simulink model "PMSM_DemoBackup"  (R2020a)
settings: Solver=FixedStepDiscrete  StartTime=0.0  StopTime=Inf  FixedStep=1000e-6  RelTol=1e-3  EnableMultiTasking=on
PreLoadFcn:
  | run('PMSM_Demo_ini.m');
PostLoadFcn:
  | , if any(exist('dsrtsu_mdlpostloadfcn', 'file') ~= 0), dsrtsu_mdlpostloadfcn('Execute', bdroot); end,
InitFcn:
  | , if any(exist('rtifpga_mdlclblib', 'file') ~= 0), rtifpga_mdlclblib('Init', bdroot); end,
undefined symbols (not defined in the file): clock, Const_Id_Fieldweakening, Const_Ld_Stator, Const_Lq_Stator, Const_PolePairs, Const_Psi, Newton, PMSM_Ctrl_Ctrl_mode_SW, PMSM_Ctrl_fRS_Set, PMSM_Ctrl_i_d_Set, PMSM_Ctrl_i_d_Stroke, PMSM_Ctrl_i_q_Set, PMSM_Ctrl_i_q_Stroke, PMSM_Ctrl_Ki_id, PMSM_Ctrl_Ki_iq, PMSM_Ctrl_Ki_n, PMSM_Ctrl_Kp_id, PMSM_Ctrl_Kp_iq, PMSM_Ctrl_Kp_n, PMSM_Ctrl_Limit_iq, PMSM_Ctrl_load_torque, PMSM_Ctrl_n_Limit, PMSM_Ctrl_n_Set, PMSM_Ctrl_n_Stroke, PMSM_Ctrl_Pos_Src, PMSM_Ctrl_TF_Id, PMSM_Ctrl_TF_Iq, PMSM_Ctrl_TF_n, PMSM_Ctrl_theta_offset, PMSM_Ctrl_v_d_Set, PMSM_Ctrl_V_DCLink_Limit, PMSM_Ctrl_v_q_Set, PMSM_Ctrl_Vel_Src, Raphson, rpm_to_rad, s, SW_Fieldweakening, T_PWM
libraries: simulink x37, rti1202lib_adc_class1 x8, dsextras x4, rtiemclib x4, rti1202lib_dio_class1 x3, ASM_ElectricComponents_lib x2, ASM_Utils_lib x1, rti1202lib_base x1
(part 2 of 4)

== system PMSM_DemoBackup/Control/Output ==
  note: a,b,c
      | a,c,b
      | b,a,c
      | b,c,a
      | c,a,b
      | c,b,a
  T_Sample[s] : Inport
  PWM_Duty[a,b,c] : Inport  Port=2
  Bus Selector : BusSelector  OutputSignals=DutyCycle[a;b;c][HSD].DutyCycle_a_HSD[0_1],DutyCycle[a;b;c][HSD].DutyCycle_b_HSD[0_1],DutyCycle[a;b;c][HSD].DutyCycle_c_HSD[0_1]
  Duty_A : Constant  Value=0
  Duty_B : Constant  Value=0
  Duty_C : Constant  Value=0
  EMC_MC_PWM_BL1 : rtiemclib/EMC_MC_PWM_BL1  DSProperties=struct('RTI',struct('Version',uint32(2),'BlockType',struct('isSLSource',uint8(0),'isSLSink',uint8(1),'isHWSource',uint8(0),'isHWSink',uint8(1),'isSetup',uint8(0),'isInline',uint8(1),'isNonInline',uint8(0),'isInterrupt',uint8(0),'isChannelwise',uint8(1)),'IOBoardType','DSEMC','UnitType','MCPWM','Identifier','MCPWM','DialogType','ML','BlockSet','RTIEMC','SlaveProcessor','NONE'))  RTIBlockInterface=struct('InputPortsWidth',int32([1 3 1]),'InputPortsActive',[1 1 0],'InputPortsName',{{'Period',['Duty Cycle'],['Output Enable']}},'BlockDisplay',{{['EMC Multi Channel PWM\nPort: 1\nChannel: 7\nNumber of channels: 3'],'center'}},'IconTransparency','on','InitLevel',3,'DialogFcn','rtiemcmcpwmgui','BlockName',struct('Token',{{'EMC_MC_PWM_BL1'}}),'InputPortsDataType',{{'SS_DOUBLE','SS_DOUBLE','SS_BOOLEAN'}})  RTIBlockParameters=struct('PortNo',{{1,'OFF',[1 3]}},'ChannelNo',{{7,'OFF',[1 16]}},'InvChannelMode',{{2,'OFF',[1 2]}},'NumOfChannels',{{3,'OFF',[1 5]}},'HighLevel',{{3,'OFF',[1 3]}},'AlignmentMode',{{1,'OFF',[1 2]}},'UpdateModeCA',{{3,'OFF',[1 3]}},'UpdateModeEA',{{1,'OFF',[1 2]}},'DeadTime',{{'0.000001','OFF',[0 0.000655]}},'InitPeriod',{{'5e-05','OFF',[1e-7 1.34]}},'InitDutyCycle1',{{'0.5','OFF',[0 1]}},'InitDutyCycle2',{{'0.5','OFF',[0 1]}},'InitDutyCycle3',{{'0.5','OFF',[0 1]}},'InitDutyCycle4',{{'0.5','OFF',[0 1]}},'InitDutyCycle5',{{'0.5','OFF',[0 1]}},'InitDutyCycle6',{{'0.5','OFF',[0 1]}},'InitDutyCycle7',{{'0','OFF',[0 1]}},'InitDutyCycle8',{{'0','OFF',[0 1]}},'InitDutyCycle9',{{'0','OFF',[0 1]}},'InitDutyCycle10',{{'0.5','OFF',[0 1]}},'InitDutyCycle11',{{'0.5','OFF',[0 1]}},'InitDutyCycle12',{{'0.5','OFF',[0 1]}},'InitDutyCycle13',{{'0.5','OFF',[0 1]}},'InitDutyCycle14',{{'0.5','OFF',[0 1]}},'InitDutyCycle15',{{'0.5','OFF',[0 1]}},'InitDutyCycle16',{{'0.5','OFF',[0 1]}},'TerminationMode',{{0,'OFF',[0 1]}},'OutputTermValidate',{{0,'OFF',[0 1]}},'TermPeriod',{{'5e-05','OFF',[1e-7 1.34]}},'TermDutyCycle1',{{'0.5','OFF',[0 1]}},'TermDutyCycle2',{{'0.5','OFF',[0 1]}},'TermDutyCycle3',{{'0.5','OFF',[0 1]}},'TermDutyCycle4',{{'0.5','OFF',[0 1]}},'TermDutyCycle5',{{'0.5','OFF',[0 1]}},'TermDutyCycle6',{{'0.5','OFF',[0 1]}},'TermDutyCycle7',{{'0.5','OFF',[0 1]}},'TermDutyCycle8',{{'0.5','OFF',[0 1]}},'TermDutyCycle9',{{'0.5','OFF',[0 1]}},'TermDutyCycle10',{{'0.5','OFF',[0 1]}},'TermDutyCycle11',{{'0.5','OFF',[0 1]}},'TermDutyCycle12',{{'0.5','OFF',[0 1]}},'TermDutyCycle13',{{'0.5','OFF',[0 1]}},'TermDutyCycle14',{{'0.5','OFF',[0 1]}},'TermDutyCycle15',{{'0.5','OFF',[0 1]}},'TermDutyCycle16',{{'0.5','OFF',[0 1]}},'EnableEvent',{{1,'OFF',[0 1]}},'EventMode',{{3,'OFF',[1 3]}},'EventOnStart',{{0,'OFF',[0 1]}},'EventOnCenter',{{1,'OFF',[0 1]}},'EventDelay',{{'0','OFF',[0 1.34]}},'EventRate',{{'1','OFF',[1 256]}},'TriggerLine',{{1,'OFF',[1 16]}},'TLCFileName',{{'rtiemcmcpwm','OFF',[]}},'ValidateDeadTimeBuildCheck',{{true,'OFF',[]}},'InitDutyCycleBuildCheck1',{{0,'OFF',[]}},'InitDutyCycleBuildCheck2',{{0,'OFF',[]}},'InitDutyCycleBuildCheck3',{{0,'OFF',[]}},'InitDutyCycleBuildCheck4',{{0,'OFF',[]}},'InitDutyCycleBuildCheck5',{{0,'OFF',[]}},'InitDutyCycleBuildCheck6',{{0,'OFF',[]}},'InitDutyCycleBuildCheck7',{{1,'OFF',[]}},'InitDutyCycleBuildCheck8',{{1,'OFF',[]}},'InitDutyCycleBuildCheck9',{{1,'OFF',[]}},'InitDutyCycleBuildCheck10',{{0,'OFF',[]}},'InitDutyCycleBuildCheck11',{{0,'OFF',[]}},'InitDutyCycleBuildCheck12',{{0,'OFF',[]}},'InitDutyCycleBuildCheck13',{{0,'OFF',[]}},'InitDutyCycleBuildCheck14',{{0,'OFF',[]}},'InitDutyCycleBuildCheck15',{{0,'OFF',[]}},'InitDutyCycleBuildCheck16',{{0,'OFF',[]}},'ValidateTermBuildCheck',{{false,'OFF',[]}},'TermDutyCycleBuildCheck1',{{0,'OFF',[]}},'TermDutyCycleBuildCheck2',{{0,'OFF',[]}},'TermDutyCycleBuildCheck3',{{0,'OFF',[]}},'TermDutyCycleBuildCheck4',{{0,'OFF',[]}},'TermDutyCycleBuildCheck5',{{0,'OFF',[]}},'TermDutyCycleBuildCheck6',{{0,'OFF',[]}},'TermDutyCycleBuildCheck7',{{0,'OFF',[]}},'TermDutyCycleBuildCheck8',{{0,'OFF',[]}},'TermDutyCycleBuildCheck9',{{0,'OFF',[]}},'TermDutyCycleBuildCheck10',{{0,'OFF',[]}},'TermDutyCycleBuildCheck11',{{0,'OFF',[]}},'TermDutyCycleBuildCheck12',{{0,'OFF',[]}},'TermDutyCycleBuildCheck13',{{0,'OFF',[]}},'TermDutyCycleBuildCheck14',{{0,'OFF',[]}},'TermDutyCycleBuildCheck15',{{0,'OFF',[]}},'TermDutyCycleBuildCheck16',{{0,'OFF',[]}},'ValidateEventBuildCheck',{{true,'OFF',[]}},'ActivateOutputEnablePort',{{0,'OFF',[0 1]}},'InitOutputEnable',{{1,'OFF',[1 2]}})  RTISFcnParameters=struct('PortNo','int32','ChannelNo','int32','InvChannelMode','int32','NumOfChannels','int32','HighLevel','int32','AlignmentMode','int32','UpdateModeCA','int32','UpdateModeEA','int32','DeadTime','double','InitPeriod','double','InitDutyCycle1','double','InitDutyCycle2','double','InitDutyCycle3','double','InitDutyCycle4','double','InitDutyCycle5','double','InitDutyCycle6','double','InitDutyCycle7','double','InitDutyCycle8','double','InitDutyCycle9','double','InitDutyCycle10','double','InitDutyCycle11','double','InitDutyCycle12','double','InitDutyCycle13','double','InitDutyCycle14','double','InitDutyCycle15','double','InitDutyCycle16','double','TerminationMode','uint32','OutputTermValidate','int32','TermPeriod','double','TermDutyCycle1','double','TermDutyCycle2','double','TermDutyCycle3','double','TermDutyCycle4','double','TermDutyCycle5','double','TermDutyCycle6','double','TermDutyCycle7','double','TermDutyCycle8','double','TermDutyCycle9','double','TermDutyCycle10','double','TermDutyCycle11','double','TermDutyCycle12','double','TermDutyCycle13','double','TermDutyCycle14','double','TermDutyCycle15','double','TermDutyCycle16','double','EnableEvent','int32','EventMode','int32','EventOnStart','int32','EventOnCenter','int32','EventDelay','double','EventRate','int32','TriggerLine','int32','TLCFileName','char','ActivateOutputEnablePort','int32','InitOutputEnable','int32')  RTIBlockParaDefault=struct('PortNo',1,'ChannelNo',1,'InvChannelMode',1,'NumOfChannels',1,'HighLevel',1,'AlignmentMode',1,'UpdateModeCA',1,'UpdateModeEA',1,'DeadTime',0,'InitPeriod',5e-5,'InitDutyCycle1',2^-1,'InitDutyCycle2',2^-1,'InitDutyCycle3',2^-1,'InitDutyCycle4',2^-1,'InitDutyCycle5',2^-1,'InitDutyCycle6',2^-1,'InitDutyCycle7',2^-1,'InitDutyCycle8',2^-1,'InitDutyCycle9',2^-1,'InitDutyCycle10',2^-1,'InitDutyCycle11',2^-1,'InitDutyCycle12',2^-1,'InitDutyCycle13',2^-1,'InitDutyCycle14',2^-1,'InitDutyCycle15',2^-1,'InitDutyCycle16',2^-1,'TerminationMode',0,'OutputTermValidate',0,'TermPeriod',5e-5,'TermDutyCycle1',2^-1,'TermDutyCycle2',2^-1,'TermDutyCycle3',2^-1,'TermDutyCycle4',2^-1,'TermDutyCycle5',2^-1,'TermDutyCycle6',2^-1,'TermDutyCycle7',2^-1,'TermDutyCycle8',2^-1,'TermDutyCycle9',2^-1,'TermDutyCycle10',2^-1,'TermDutyCycle11',2^-1,'TermDutyCycle12',2^-1,'TermDutyCycle13',2^-1,'TermDutyCycle14',2^-1,'TermDutyCycle15',2^-1,'TermDutyCycle16',2^-1,'EnableEvent',0,'EventMode',1,'EventOnStart',1,'EventOnCenter',0,'EventDelay',0,'EventRate',1,'TriggerLine',1,'TLCFileName','rtiemcmcpwm','ValidateDeadTimeBuildCheck',0,'InitDutyCycleBuildCheck1',0,'InitDutyCycleBuildCheck2',0,'InitDutyCycleBuildCheck3',0,'InitDutyCycleBuildCheck4',0,'InitDutyCycleBuildCheck5',0,'InitDutyCycleBuildCheck6',0,'InitDutyCycleBuildCheck7',0,'InitDutyCycleBuildCheck8',0,'InitDutyCycleBuildCheck9',0,'InitDutyCycleBuildCheck10',0,'InitDutyCycleBuildCheck11',0,'InitDutyCycleBuildCheck12',0,'InitDutyCycleBuildCheck13',0,'InitDutyCycleBuildCheck14',0,'InitDutyCycleBuildCheck15',0,'InitDutyCycleBuildCheck16',0,'ValidateTermBuildCheck',0,'TermDutyCycleBuildCheck1',0,'TermDutyCycleBuildCheck2',0,'TermDutyCycleBuildCheck3',0,'TermDutyCycleBuildCheck4',0,'TermDutyCycleBuildCheck5',0,'TermDutyCycleBuildCheck6',0,'TermDutyCycleBuildCheck7',0,'TermDutyCycleBuildCheck8',0,'TermDutyCycleBuildCheck9',0,'TermDutyCycleBuildCheck10',0,'TermDutyCycleBuildCheck11',0,'TermDutyCycleBuildCheck12',0,'TermDutyCycleBuildCheck13',0,'TermDutyCycleBuildCheck14',0,'TermDutyCycleBuildCheck15',0,'TermDutyCycleBuildCheck16',0,'ValidateEventBuildCheck',0,'ActivateOutputEnablePort',0,'InitOutputEnable',1)
      settings: SourceProductName=dSPACE RTI Electric Motor Control Blockset
  Mux : Mux  Inputs=3
  Mux1 : Mux  Inputs=3
  Switch : Switch  Criteria=u2 ~= 0
  UseController : Constant
  wires:
  PWM_Duty[a,b,c]/1 -> Bus Selector/1
  T_Sample[s]/1 -> EMC_MC_PWM_BL1/1
  Bus Selector/1 -> Mux/1  "<DutyCycle_a_HSD[0_1]>"
  Bus Selector/2 -> Mux/2  "<DutyCycle_b_HSD[0_1]>"
  Bus Selector/3 -> Mux/3  "<DutyCycle_c_HSD[0_1]>"
  Duty_A/1 -> Mux1/1
  Duty_C/1 -> Mux1/3
  Duty_B/1 -> Mux1/2
  Switch/1 -> EMC_MC_PWM_BL1/2
  Mux/1 -> Switch/1
  Mux1/1 -> Switch/3
  UseController/1 -> Switch/2

== system PMSM_DemoBackup/Control/pmsm_ctrl_par_sig ==
  rect_pulse : Inport
  MDL_DISP : Subsystem
      mask Display: disp('Simulation results:\nArbitrary input to\nControlDesk from MDL')
  MDL_DISP_INPUT : Subsystem
      mask Display: disp('Simulation results:\nArbitrary input to\nControlDesk from MDL')
  MDL_PAR : Subsystem
      mask Display: disp('Simulation parameters:\nContinuous output from\nControlDesk to MDL')
  wires:
  rect_pulse/1 -> MDL_PAR/1(rect_pulse)

== system PMSM_DemoBackup/RTI Data/RTI Data Store ==
  RTI Data Store : Subsystem  mask(RTI_DATA_STORE){}
      mask help:
      | RTI Data Store Block. This block is used by RTI to store internal model dependent data. Deleting this block will result in data loss.
      |
      | NEVER DELETE, COPY, OR MODIFY THIS BLOCK!
      mask Help:
      | RTI Data Store Block. This block is used by RTI to store internal model dependent data. Deleting this block will result in data loss.
      | 
      | NEVER DELETE, COPY, OR MODIFY THIS BLOCK!
      mask Display: text(0.5, 0.5, ' ', 'HorizontalAlignment', 'center');

== system PMSM_DemoBackup/Ref_value_gen/Enabled and Triggered Subsystem ==
  n_ref : Inport
  Constant : Constant
  Constant1 : Constant  Value=0
  Hit Crossing : HitCross  HitCrossingOffset=0.5  HitCrossingDirection=rising
  Memory : Memory  InheritSampleTime=on
  Product : Product  RndMeth=Zero
  Relational Operator : RelationalOperator  Operator=<=  OutDataTypeStr=boolean  RndMeth=Nearest
  Relational Operator1 : RelationalOperator  OutDataTypeStr=boolean  RndMeth=Nearest
  Sum : Sum  Inputs=|++
  Switch : Switch  Threshold=0.5
  Switch1 : Switch  Threshold=0.5
  load_signal_0 : Constant  Value=0
  load_signal_generator : Constant
  start_time_samples : Constant  Value=1000
  switch_out_boarder : Constant  Value=0.5
  load_ref : Outport  VectorParamsAs1DForOutWhenUnconnected=off
  wires:
  Constant/1 -> Sum/1
  Sum/1 -> Switch/3
  Constant1/1 -> Switch/1
  Switch/1 -> Relational Operator/1, Memory/1
  Hit Crossing/1 -> Switch/2
  n_ref/1 -> Hit Crossing/1, Relational Operator1/1
  start_time_samples/1 -> Relational Operator/2
  load_signal_0/1 -> Switch1/1
  Relational Operator/1 -> Switch1/2
  load_signal_generator/1 -> Switch1/3
  Switch1/1 -> Product/2
  switch_out_boarder/1 -> Relational Operator1/2
  Product/1 -> load_ref/1
  Relational Operator1/1 -> Product/1
  Memory/1 -> Sum/2

== system PMSM_DemoBackup/Control/Control_load_machine/duty_cycle_2_torque ==
  In_duty_cycle[0..1] : Inport
  Divide : Product  Inputs=*/
  coil_resistance : Constant  Value=24
  current_2_load1 : Lookup_n-D  NumberOfTableDimensions=1  BreakpointsForDimension1=[0, 0.05, 0.1, 0.2, 0.3, 0.4]  Table=[0, 0.05, 0.2, 0.7, 1.4, 1.9]  InputSameDT=on
  duty_cycle_2_voltage : Subsystem
  Out_torque[Nm] : Outport  VectorParamsAs1DForOutWhenUnconnected=off
  wires:
  In_duty_cycle[0..1]/1 -> duty_cycle_2_voltage/1(In_duty_cycle[0..1])
  duty_cycle_2_voltage/1(Out_duty_voltage[V]) -> Divide/1
  coil_resistance/1 -> Divide/2
  current_2_load1/1 -> Out_torque[Nm]/1
  Divide/1 -> current_2_load1/1

== system PMSM_DemoBackup/Control/Control_load_machine/torque_2_duty_cycle ==
  In_torque[Nm] : Inport
  current_2_voltage : Gain  Gain=24
  load_2_current4 : Lookup_n-D  NumberOfTableDimensions=1  BreakpointsForDimension1=[0, 0.05, 0.2, 0.7, 1.4, 1.9]  Table=[0, 0.05, 0.1, 0.2, 0.3, 0.4]  InputSameDT=on
  voltage_2_duty_cycle : Subsystem
  Out_duty_cycle[0..1] : Outport  VectorParamsAs1DForOutWhenUnconnected=off
  wires:
  load_2_current4/1 -> current_2_voltage/1
  current_2_voltage/1 -> voltage_2_duty_cycle/1(In_voltage[V])
  In_torque[Nm]/1 -> load_2_current4/1
  voltage_2_duty_cycle/1(Out_duty_cycle) -> Out_duty_cycle[0..1]/1

== system PMSM_DemoBackup/Control/Control_load_machine/torque_2_duty_cycle1 ==
  In_torque[Nm] : Inport
  current_2_voltage : Gain  Gain=24
  load_2_current4 : Lookup_n-D  NumberOfTableDimensions=1  BreakpointsForDimension1=[0, 0.05, 0.2, 0.7, 1.4, 1.9]  Table=[0, 0.05, 0.1, 0.2, 0.3, 0.4]  InputSameDT=on
  voltage_2_duty_cycle : Subsystem
  Out_duty_cycle[0..1] : Outport  VectorParamsAs1DForOutWhenUnconnected=off
  wires:
  voltage_2_duty_cycle/1(Out_duty_cycle[0..1]) -> Out_duty_cycle[0..1]/1
  In_torque[Nm]/1 -> load_2_current4/1
  current_2_voltage/1 -> voltage_2_duty_cycle/1(In_voltage[V])
  load_2_current4/1 -> current_2_voltage/1

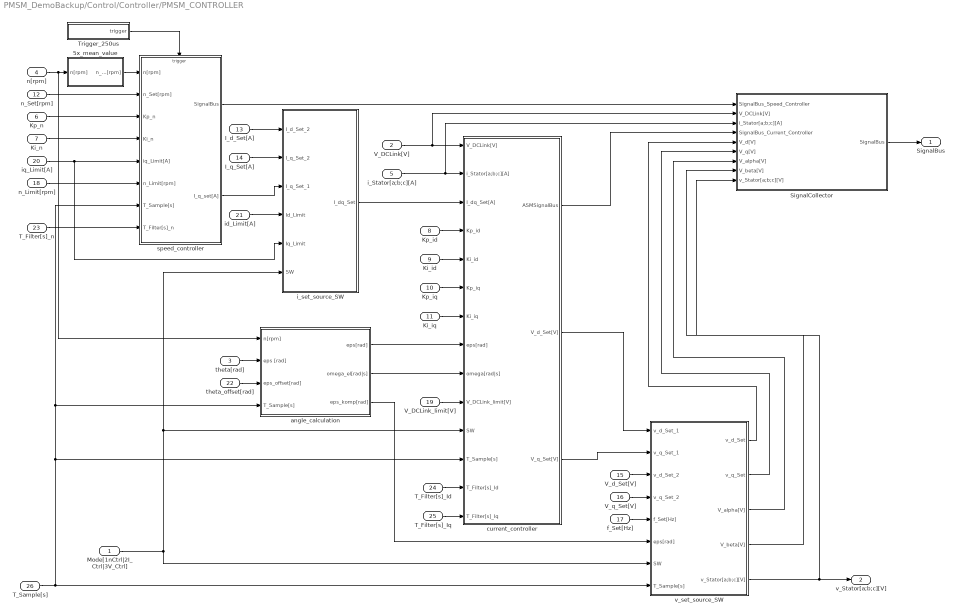
== system PMSM_DemoBackup/Control/Controller/PMSM_CONTROLLER ==
  Mode[1nCtrl|2I_Ctrl|3V_Ctrl] : Inport
  V_DCLink[V] : Inport  Port=2
  theta[rad] : Inport  Port=3
  n[rpm] : Inport  Port=4
  i_Stator[a;b;c][A] : Inport  Port=5
  Kp_n : Inport  Port=6
  Ki_n : Inport  Port=7
  Kp_id : Inport  Port=8
  Ki_id : Inport  Port=9
  Kp_iq : Inport  Port=10
  Ki_iq : Inport  Port=11
  n_Set[rpm] : Inport  Port=12
  I_d_Set[A] : Inport  Port=13
  I_q_Set[A] : Inport  Port=14
  V_d_Set[V] : Inport  Port=15
  V_q_Set[V] : Inport  Port=16
  f_Set[Hz] : Inport  Port=17
  n_Limit[rpm] : Inport  Port=18
  V_DCLink_limit[V] : Inport  Port=19
  iq_Limit[A] : Inport  Port=20
  id_Limit[A] : Inport  Port=21
  theta_offset[rad] : Inport  Port=22
  T_Filter[s]_n : Inport  Port=23
  T_Filter[s]_Id : Inport  Port=24
  T_Filter[s]_Iq : Inport  Port=25
  T_Sample[s] : Inport  Port=26
  5x_mean_value : Subsystem
  SignalCollector : Subsystem
  Trigger_250us : Subsystem
  angle_calculation : Subsystem
  current_controller : Subsystem
  i_set_source_SW : Subsystem
  speed_controller : Subsystem
  v_set_source_SW : Subsystem
  SignalBus : Outport  VectorParamsAs1DForOutWhenUnconnected=off
  v_Stator[a;b;c][V] : Outport  Port=2  VectorParamsAs1DForOutWhenUnconnected=off
  wires:
  current_controller/3(" V_q_Set[V]") -> v_set_source_SW/2(v_q_Set_1)
  v_set_source_SW/2(v_q_Set) -> SignalCollector/6(V_q[V])
  v_set_source_SW/1(v_d_Set) -> SignalCollector/5(V_d[V])
  i_Stator[a;b;c][A]/1 -> current_controller/2(i_Stator[a;b;c][A]), SignalCollector/3(i_Stator[a;b;c][A])
  T_Sample[s]/1 -> v_set_source_SW/8(T_Sample[s]), current_controller/12(T_Sample[s]), speed_controller/7(T_Sample[s]), angle_calculation/4(T_Sample[s])
  id_Limit[A]/1 -> i_set_source_SW/4(Id_Limit)
  speed_controller/1(SignalBus) -> SignalCollector/1(SignalBus_Speed_Controller)
  angle_calculation/1(eps[rad]) -> current_controller/8(eps[rad])
  current_controller/2(" V_d_Set[V]") -> v_set_source_SW/1(v_d_Set_1)
  V_DCLink[V]/1 -> current_controller/1(V_DCLink[V]), SignalCollector/2(V_DCLink[V])
  i_set_source_SW/1(I_dq_Set) -> current_controller/3(I_dq_Set[A])
  current_controller/1(ASMSignalBus) -> SignalCollector/4(SignalBus_Current_Controller)
  angle_calculation/2(omega_el[rad|s]) -> current_controller/9(omega[rad|s])
  theta[rad]/1 -> angle_calculation/2(eps [rad])
  V_q_Set[V]/1 -> v_set_source_SW/4(v_q_Set_2)
  V_d_Set[V]/1 -> v_set_source_SW/3(v_d_Set_2)
  Mode[1nCtrl|2I_Ctrl|3V_Ctrl]/1 -> v_set_source_SW/7(SW), i_set_source_SW/6(SW), current_controller/11(SW)
  SignalCollector/1(SignalBus) -> SignalBus/1
  v_set_source_SW/5(v_Stator[a;b;c][V]) -> SignalCollector/9(v_Stator[a;b;c][V]), v_Stator[a;b;c][V]/1
  f_Set[Hz]/1 -> v_set_source_SW/5(f_Set[Hz])
  theta_offset[rad]/1 -> angle_calculation/3(eps_offset[rad])
  angle_calculation/3(eps_komp[rad]) -> v_set_source_SW/6(eps[rad])
  Kp_id/1 -> current_controller/4(Kp_id)
  Ki_id/1 -> current_controller/5(Ki_id)
  Kp_iq/1 -> current_controller/6(Kp_iq)
  Ki_iq/1 -> current_controller/7(Ki_iq)
  V_DCLink_limit[V]/1 -> current_controller/10(V_DCLink_limit[V])
  I_d_Set[A]/1 -> i_set_source_SW/1(I_d_Set_2)
  I_q_Set[A]/1 -> i_set_source_SW/2(I_q_Set_2)
  speed_controller/2(I_q_set[A]) -> i_set_source_SW/3(I_q_Set_1)
  n_Set[rpm]/1 -> speed_controller/2(n_Set[rpm])
  n[rpm]/1 -> angle_calculation/1(n[rpm]), 5x_mean_value/1(n[rpm])
  iq_Limit[A]/1 -> i_set_source_SW/5(Iq_Limit), speed_controller/5(iq_Limit[A])
  n_Limit[rpm]/1 -> speed_controller/6(n_Limit[rpm])
  Kp_n/1 -> speed_controller/3(Kp_n)
  Ki_n/1 -> speed_controller/4(Ki_n)
  T_Filter[s]_n/1 -> speed_controller/8(T_Filter[s]_n)
  T_Filter[s]_Id/1 -> current_controller/13(T_Filter[s]_Id)
  T_Filter[s]_Iq/1 -> current_controller/14(T_Filter[s]_Iq)
  v_set_source_SW/3(V_alpha[V]) -> SignalCollector/7(V_alpha[V])
  v_set_source_SW/4(V_beta[V]) -> SignalCollector/8(V_beta[V])
  5x_mean_value/1(n_mean[rpm]) -> speed_controller/1(n[rpm])
  Trigger_250us/1(trigger) -> speed_controller/Trigger

== system PMSM_DemoBackup/Control/Controller/SPACE_VECTOR_MODULATOR ==
  V_DCLink[V] : Inport
  v_Stator[a;b;c][V] : Inport  Port=2
  Label_DutyCycle_HSD[a;b;c][0_1] : Subsystem
  Label_DutyCycle_LSD[a;b;c][0_1] : Subsystem
  Max : MinMax  Function=max  InputSameDT=on  SaturateOnIntegerOverflow=on
  Min : MinMax  InputSameDT=on  SaturateOnIntegerOverflow=on
  Product : Product  Inputs=*/  SaturateOnIntegerOverflow=on  OutDataTypeStr=Inherit: Same as first input
  Saturation : Saturate  UpperLimit=1  LowerLimit=0
  SignalCollector : Subsystem
  Sum : Sum  Inputs=+-|  SaturateOnIntegerOverflow=on
  Sum2 : Sum  Inputs=-++  SaturateOnIntegerOverflow=on
  Sum3 : Sum  Inputs=-+|  SaturateOnIntegerOverflow=on
  Sum4 : Sum  Inputs=-+|  SaturateOnIntegerOverflow=on
  half : Gain  Gain=1/2  SaturateOnIntegerOverflow=on  OutDataTypeStr=Inherit: Same as input  ParamDataTypeStr=Inherit: Same as input
  one : Constant
  SignalBus : Outport  VectorParamsAs1DForOutWhenUnconnected=off
  DutyCycle_HSD[a;b;c][0_1] : Outport  Port=2  VectorParamsAs1DForOutWhenUnconnected=off
  DutyCycle_LSD[a;b;c][0_1] : Outport  Port=3  VectorParamsAs1DForOutWhenUnconnected=off
  wires:
  Sum3/1 -> Label_DutyCycle_LSD[a;b;c][0_1]/1(In)
  Min/1 -> Sum/2, Sum2/1
  Max/1 -> Sum/1
  Sum4/1 -> half/1
  Sum/1 -> Sum4/1
  one/1 -> Sum4/2, Sum3/2
  Sum2/1 -> Saturation/1
  Saturation/1 -> Sum3/1, Label_DutyCycle_HSD[a;b;c][0_1]/1(In)
  V_DCLink[V]/1 -> Product/2
  v_Stator[a;b;c][V]/1 -> Product/1
  half/1 -> Sum2/3
  Product/1 -> Sum2/2, Max/1, Min/1
  Label_DutyCycle_LSD[a;b;c][0_1]/1(Out) -> DutyCycle_LSD[a;b;c][0_1]/1, SignalCollector/2(DutyCycle_LSD[a;b;c][0_1])
  Label_DutyCycle_HSD[a;b;c][0_1]/1(Out) -> DutyCycle_HSD[a;b;c][0_1]/1, SignalCollector/1(DutyCycle_HSD[a;b;c][0_1])
  SignalCollector/1(SignalBus) -> SignalBus/1

== system PMSM_DemoBackup/Control/Controller/SignalCollector ==
  BusCreator : BusCreator  Inputs=1
  tag scope: BUS_PMSM_Ctrl=global
  wires:
  [BUS_PMSM_CONTROLLER] -> BusCreator/1
  BusCreator/1 -> [BUS_PMSM_Ctrl]  "PMSM_Ctrl"

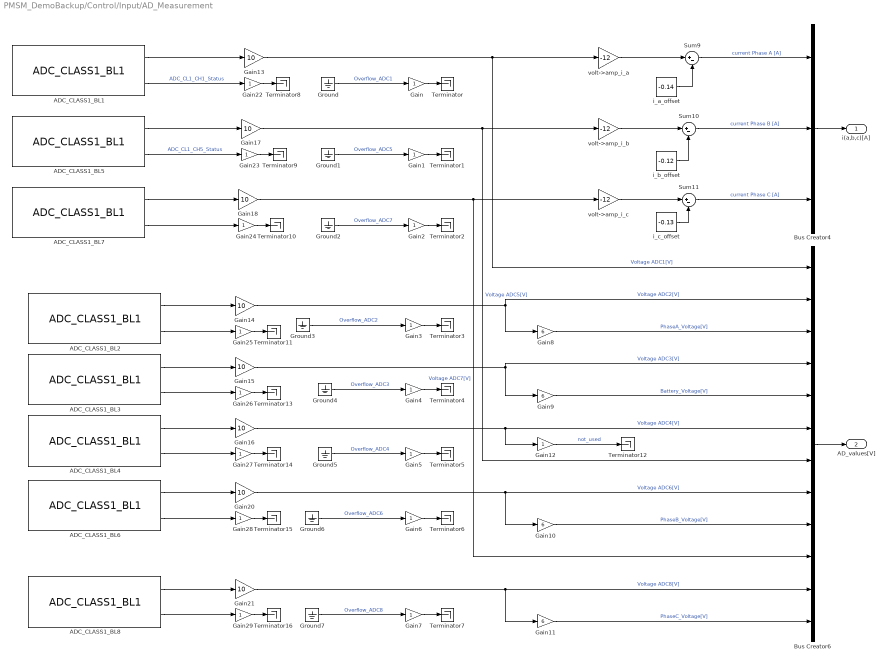
== system PMSM_DemoBackup/Control/Input/AD_Measurement ==
  " i_a_offset" : Constant  Value=-0.14
  " i_b_offset  " : Constant  Value=-0.12
  ADC_CLASS1_BL1 : rti1202lib_adc_class1/ADC_CLASS1_BL1  DSProperties=struct('RTI',struct('Version',uint32(1),'BlockType',struct('isSLSource',uint8(1),'isSLSink',uint8(1),'isHWSource',uint8(0),'isHWSink',uint8(1),'isSetup',uint8(0),'isInline',uint8(1),'isNonInline',uint8(0),'isInterrupt',uint8(0),'isChannelwise',uint8(1)),'IOBoardType',{{'DS120X','STD','ADCC1'}},'UnitType','ADC','Identifier','ADC','DialogType','ML','BlockSet','NONE','SlaveProcessor','NONE'))  RTIBlockInterface=struct('InputPortsActive',0,'InputPortsWidth',int32(1),'InputPortsDataType',{{'SS_BOOLEAN'}},'InputPortsName',{{'Continue'}},'OutputPortsActive',[1 1],'OutputPortsWidth',int32([1 1]),'OutputPortsDataType',{{'SS_DOUBLE','SS_INT16'}},'OutputPortsName',{{'ADC','Status'}},'DialogFcn','rti120xstdadcc1adcgui','SampleTime',{{-1}},'InitLevel',3,'IconTransparency','on','BlockDisplay',{{['ADC CL1\nChannel: 1'],'center'}},'BlockName',struct('Token',{{'ADC_CLASS1_BL1'}}))  RTIBlockParameters=struct('ReadMode',{{2,'OFF',[1 2]}},'ChannelNo',{{1,'OFF',[]}},'ConversionMode',{{1,'OFF',[1 2]}},'TriggerSource',{{2,'OFF',[1 2]}},'TriggerLineIn',{{1,'OFF',[1 16]}},'SampleMode',{{1,'OFF',[1 2]}},'BurstTriggerSource',{{1,'OFF',[1 2]}},'BurstTriggerLine',{{1,'OFF',[1 16]}},'ConvTriggerSource',{{3,'OFF',[1 3]}},'ConvTriggerLine',{{1,'OFF',[1 16]}},'ConvPeriod',{{'100e-6','OFF',[1e-6 1.34]}},'ConvPeriodCheck',{{0,'OFF',[]}},'BurstSize',{{'10','OFF',[]}},'BurstSizeCheck',{{0,'OFF',[]}},'DataSetOffset',{{'0','OFF',[]}},'DataSetOffsetCheck',{{0,'OFF',[]}},'DataSetLength',{{'1','OFF',[]}},'DataSetLengthCheck',{{0,'OFF',[]}},'EnableTriggerEvent',{{0,'OFF',[0 1]}},'TriggerMode',{{2,'OFF',[1 3]}},'TriggerLineOut',{{1,'OFF',[1 16]}},'ADCSWStartEnable',{{0,'OFF',[0 1]}},'SampleTime',{{'-1','OFF',[-1 inf]}},'SampleTimeCheck',{{0,'OFF',[]}},'StatusPortEnable',{{1,'OFF',[0 1]}},'TLCFileName',{{'rti120xadc_c1_adc','OFF',[]}})  RTISFcnParameters=struct('ReadMode','int16','ChannelNo','int16','ConversionMode','int16','TriggerSource','int16','TriggerLineIn','int16','SampleMode','int16','BurstTriggerSource','int16','BurstTriggerLine','int16','ConvTriggerSource','int16','ConvTriggerLine','int16','ConvPeriod','double','BurstSize','int16','DataSetOffset','int16','DataSetLength','int16','EnableTriggerEvent','int16','TriggerMode','int16','TriggerLineOut','int16','ADCSWStartEnable','int16','SampleTime','double','StatusPortEnable','int16','TLCFileName','char')  RTIBlockParaDefault=struct('ReadMode',1,'ChannelNo',1,'ConversionMode',1,'TriggerSource',1,'TriggerLineIn',1,'SampleMode',1,'BurstTriggerSource',1,'BurstTriggerLine',1,'ConvTriggerSource',3,'ConvTriggerLine',1,'ConvPeriod',0.0001,'ConvPeriodCheck',0,'BurstSize',10,'BurstSizeCheck',0,'DataSetOffset',0,'DataSetOffsetCheck',0,'DataSetLength',1,'DataSetLengthCheck',0,'EnableTriggerEvent',0,'TriggerMode',2,'TriggerLineOut',1,'ADCSWStartEnable',0,'SampleTime',-1,'SampleTimeCheck',1,'StatusPortEnable',0,'TLCFileName','rti120xadc_c1_adc')
  ADC_CLASS1_BL2 : rti1202lib_adc_class1/ADC_CLASS1_BL1  DSProperties=struct('RTI',struct('Version',uint32(1),'BlockType',struct('isSLSource',uint8(1),'isSLSink',uint8(1),'isHWSource',uint8(0),'isHWSink',uint8(1),'isSetup',uint8(0),'isInline',uint8(1),'isNonInline',uint8(0),'isInterrupt',uint8(0),'isChannelwise',uint8(1)),'IOBoardType',{{'DS120X','STD','ADCC1'}},'UnitType','ADC','Identifier','ADC','DialogType','ML','BlockSet','NONE','SlaveProcessor','NONE'))  RTIBlockInterface=struct('InputPortsActive',0,'InputPortsWidth',int32(1),'InputPortsDataType',{{'SS_BOOLEAN'}},'InputPortsName',{{'Continue'}},'OutputPortsActive',[1 1],'OutputPortsWidth',int32([1 1]),'OutputPortsDataType',{{'SS_DOUBLE','SS_INT16'}},'OutputPortsName',{{'ADC','Status'}},'DialogFcn','rti120xstdadcc1adcgui','SampleTime',{{-1}},'InitLevel',3,'IconTransparency','on','BlockDisplay',{{['ADC CL1\nChannel: 2'],'center'}},'BlockName',struct('Token',{{'ADC_CLASS1_BL1'}}))  RTIBlockParameters=struct('ReadMode',{{2,'OFF',[1 2]}},'ChannelNo',{{2,'OFF',[]}},'ConversionMode',{{1,'OFF',[1 2]}},'TriggerSource',{{2,'OFF',[1 2]}},'TriggerLineIn',{{1,'OFF',[1 16]}},'SampleMode',{{1,'OFF',[1 2]}},'BurstTriggerSource',{{1,'OFF',[1 2]}},'BurstTriggerLine',{{1,'OFF',[1 16]}},'ConvTriggerSource',{{3,'OFF',[1 3]}},'ConvTriggerLine',{{1,'OFF',[1 16]}},'ConvPeriod',{{'100e-6','OFF',[1e-6 1.34]}},'ConvPeriodCheck',{{0,'OFF',[]}},'BurstSize',{{'10','OFF',[]}},'BurstSizeCheck',{{0,'OFF',[]}},'DataSetOffset',{{'0','OFF',[]}},'DataSetOffsetCheck',{{0,'OFF',[]}},'DataSetLength',{{'1','OFF',[]}},'DataSetLengthCheck',{{0,'OFF',[]}},'EnableTriggerEvent',{{0,'OFF',[0 1]}},'TriggerMode',{{2,'OFF',[1 3]}},'TriggerLineOut',{{1,'OFF',[1 16]}},'ADCSWStartEnable',{{0,'OFF',[0 1]}},'SampleTime',{{'-1','OFF',[-1 inf]}},'SampleTimeCheck',{{0,'OFF',[]}},'StatusPortEnable',{{1,'OFF',[0 1]}},'TLCFileName',{{'rti120xadc_c1_adc','OFF',[]}})  RTISFcnParameters=struct('ReadMode','int16','ChannelNo','int16','ConversionMode','int16','TriggerSource','int16','TriggerLineIn','int16','SampleMode','int16','BurstTriggerSource','int16','BurstTriggerLine','int16','ConvTriggerSource','int16','ConvTriggerLine','int16','ConvPeriod','double','BurstSize','int16','DataSetOffset','int16','DataSetLength','int16','EnableTriggerEvent','int16','TriggerMode','int16','TriggerLineOut','int16','ADCSWStartEnable','int16','SampleTime','double','StatusPortEnable','int16','TLCFileName','char')  RTIBlockParaDefault=struct('ReadMode',1,'ChannelNo',1,'ConversionMode',1,'TriggerSource',1,'TriggerLineIn',1,'SampleMode',1,'BurstTriggerSource',1,'BurstTriggerLine',1,'ConvTriggerSource',3,'ConvTriggerLine',1,'ConvPeriod',0.0001,'ConvPeriodCheck',0,'BurstSize',10,'BurstSizeCheck',0,'DataSetOffset',0,'DataSetOffsetCheck',0,'DataSetLength',1,'DataSetLengthCheck',0,'EnableTriggerEvent',0,'TriggerMode',2,'TriggerLineOut',1,'ADCSWStartEnable',0,'SampleTime',-1,'SampleTimeCheck',1,'StatusPortEnable',0,'TLCFileName','rti120xadc_c1_adc')
  ADC_CLASS1_BL3 : rti1202lib_adc_class1/ADC_CLASS1_BL1  DSProperties=struct('RTI',struct('Version',uint32(1),'BlockType',struct('isSLSource',uint8(1),'isSLSink',uint8(1),'isHWSource',uint8(0),'isHWSink',uint8(1),'isSetup',uint8(0),'isInline',uint8(1),'isNonInline',uint8(0),'isInterrupt',uint8(0),'isChannelwise',uint8(1)),'IOBoardType',{{'DS120X','STD','ADCC1'}},'UnitType','ADC','Identifier','ADC','DialogType','ML','BlockSet','NONE','SlaveProcessor','NONE'))  RTIBlockInterface=struct('InputPortsActive',0,'InputPortsWidth',int32(1),'InputPortsDataType',{{'SS_BOOLEAN'}},'InputPortsName',{{'Continue'}},'OutputPortsActive',[1 1],'OutputPortsWidth',int32([1 1]),'OutputPortsDataType',{{'SS_DOUBLE','SS_INT16'}},'OutputPortsName',{{'ADC','Status'}},'DialogFcn','rti120xstdadcc1adcgui','SampleTime',{{-1}},'InitLevel',3,'IconTransparency','on','BlockDisplay',{{['ADC CL1\nChannel: 3'],'center'}},'BlockName',struct('Token',{{'ADC_CLASS1_BL1'}}))  RTIBlockParameters=struct('ReadMode',{{2,'OFF',[1 2]}},'ChannelNo',{{3,'OFF',[]}},'ConversionMode',{{1,'OFF',[1 2]}},'TriggerSource',{{2,'OFF',[1 2]}},'TriggerLineIn',{{1,'OFF',[1 16]}},'SampleMode',{{1,'OFF',[1 2]}},'BurstTriggerSource',{{1,'OFF',[1 2]}},'BurstTriggerLine',{{1,'OFF',[1 16]}},'ConvTriggerSource',{{3,'OFF',[1 3]}},'ConvTriggerLine',{{1,'OFF',[1 16]}},'ConvPeriod',{{'100e-6','OFF',[1e-6 1.34]}},'ConvPeriodCheck',{{0,'OFF',[]}},'BurstSize',{{'10','OFF',[]}},'BurstSizeCheck',{{0,'OFF',[]}},'DataSetOffset',{{'0','OFF',[]}},'DataSetOffsetCheck',{{0,'OFF',[]}},'DataSetLength',{{'1','OFF',[]}},'DataSetLengthCheck',{{0,'OFF',[]}},'EnableTriggerEvent',{{0,'OFF',[0 1]}},'TriggerMode',{{2,'OFF',[1 3]}},'TriggerLineOut',{{1,'OFF',[1 16]}},'ADCSWStartEnable',{{0,'OFF',[0 1]}},'SampleTime',{{'-1','OFF',[-1 inf]}},'SampleTimeCheck',{{0,'OFF',[]}},'StatusPortEnable',{{1,'OFF',[0 1]}},'TLCFileName',{{'rti120xadc_c1_adc','OFF',[]}})  RTISFcnParameters=struct('ReadMode','int16','ChannelNo','int16','ConversionMode','int16','TriggerSource','int16','TriggerLineIn','int16','SampleMode','int16','BurstTriggerSource','int16','BurstTriggerLine','int16','ConvTriggerSource','int16','ConvTriggerLine','int16','ConvPeriod','double','BurstSize','int16','DataSetOffset','int16','DataSetLength','int16','EnableTriggerEvent','int16','TriggerMode','int16','TriggerLineOut','int16','ADCSWStartEnable','int16','SampleTime','double','StatusPortEnable','int16','TLCFileName','char')  RTIBlockParaDefault=struct('ReadMode',1,'ChannelNo',1,'ConversionMode',1,'TriggerSource',1,'TriggerLineIn',1,'SampleMode',1,'BurstTriggerSource',1,'BurstTriggerLine',1,'ConvTriggerSource',3,'ConvTriggerLine',1,'ConvPeriod',0.0001,'ConvPeriodCheck',0,'BurstSize',10,'BurstSizeCheck',0,'DataSetOffset',0,'DataSetOffsetCheck',0,'DataSetLength',1,'DataSetLengthCheck',0,'EnableTriggerEvent',0,'TriggerMode',2,'TriggerLineOut',1,'ADCSWStartEnable',0,'SampleTime',-1,'SampleTimeCheck',1,'StatusPortEnable',0,'TLCFileName','rti120xadc_c1_adc')
  ADC_CLASS1_BL4 : rti1202lib_adc_class1/ADC_CLASS1_BL1  DSProperties=struct('RTI',struct('Version',uint32(1),'BlockType',struct('isSLSource',uint8(1),'isSLSink',uint8(1),'isHWSource',uint8(0),'isHWSink',uint8(1),'isSetup',uint8(0),'isInline',uint8(1),'isNonInline',uint8(0),'isInterrupt',uint8(0),'isChannelwise',uint8(1)),'IOBoardType',{{'DS120X','STD','ADCC1'}},'UnitType','ADC','Identifier','ADC','DialogType','ML','BlockSet','NONE','SlaveProcessor','NONE'))  RTIBlockInterface=struct('InputPortsActive',0,'InputPortsWidth',int32(1),'InputPortsDataType',{{'SS_BOOLEAN'}},'InputPortsName',{{'Continue'}},'OutputPortsActive',[1 1],'OutputPortsWidth',int32([1 1]),'OutputPortsDataType',{{'SS_DOUBLE','SS_INT16'}},'OutputPortsName',{{'ADC','Status'}},'DialogFcn','rti120xstdadcc1adcgui','SampleTime',{{-1}},'InitLevel',3,'IconTransparency','on','BlockDisplay',{{['ADC CL1\nChannel: 4'],'center'}},'BlockName',struct('Token',{{'ADC_CLASS1_BL1'}}))  RTIBlockParameters=struct('ReadMode',{{2,'OFF',[1 2]}},'ChannelNo',{{4,'OFF',[]}},'ConversionMode',{{1,'OFF',[1 2]}},'TriggerSource',{{2,'OFF',[1 2]}},'TriggerLineIn',{{1,'OFF',[1 16]}},'SampleMode',{{1,'OFF',[1 2]}},'BurstTriggerSource',{{1,'OFF',[1 2]}},'BurstTriggerLine',{{1,'OFF',[1 16]}},'ConvTriggerSource',{{3,'OFF',[1 3]}},'ConvTriggerLine',{{1,'OFF',[1 16]}},'ConvPeriod',{{'100e-6','OFF',[1e-6 1.34]}},'ConvPeriodCheck',{{0,'OFF',[]}},'BurstSize',{{'10','OFF',[]}},'BurstSizeCheck',{{0,'OFF',[]}},'DataSetOffset',{{'0','OFF',[]}},'DataSetOffsetCheck',{{0,'OFF',[]}},'DataSetLength',{{'1','OFF',[]}},'DataSetLengthCheck',{{0,'OFF',[]}},'EnableTriggerEvent',{{0,'OFF',[0 1]}},'TriggerMode',{{2,'OFF',[1 3]}},'TriggerLineOut',{{1,'OFF',[1 16]}},'ADCSWStartEnable',{{0,'OFF',[0 1]}},'SampleTime',{{'-1','OFF',[-1 inf]}},'SampleTimeCheck',{{0,'OFF',[]}},'StatusPortEnable',{{1,'OFF',[0 1]}},'TLCFileName',{{'rti120xadc_c1_adc','OFF',[]}})  RTISFcnParameters=struct('ReadMode','int16','ChannelNo','int16','ConversionMode','int16','TriggerSource','int16','TriggerLineIn','int16','SampleMode','int16','BurstTriggerSource','int16','BurstTriggerLine','int16','ConvTriggerSource','int16','ConvTriggerLine','int16','ConvPeriod','double','BurstSize','int16','DataSetOffset','int16','DataSetLength','int16','EnableTriggerEvent','int16','TriggerMode','int16','TriggerLineOut','int16','ADCSWStartEnable','int16','SampleTime','double','StatusPortEnable','int16','TLCFileName','char')  RTIBlockParaDefault=struct('ReadMode',1,'ChannelNo',1,'ConversionMode',1,'TriggerSource',1,'TriggerLineIn',1,'SampleMode',1,'BurstTriggerSource',1,'BurstTriggerLine',1,'ConvTriggerSource',3,'ConvTriggerLine',1,'ConvPeriod',0.0001,'ConvPeriodCheck',0,'BurstSize',10,'BurstSizeCheck',0,'DataSetOffset',0,'DataSetOffsetCheck',0,'DataSetLength',1,'DataSetLengthCheck',0,'EnableTriggerEvent',0,'TriggerMode',2,'TriggerLineOut',1,'ADCSWStartEnable',0,'SampleTime',-1,'SampleTimeCheck',1,'StatusPortEnable',0,'TLCFileName','rti120xadc_c1_adc')
  ADC_CLASS1_BL5 : rti1202lib_adc_class1/ADC_CLASS1_BL1  DSProperties=struct('RTI',struct('Version',uint32(1),'BlockType',struct('isSLSource',uint8(1),'isSLSink',uint8(1),'isHWSource',uint8(0),'isHWSink',uint8(1),'isSetup',uint8(0),'isInline',uint8(1),'isNonInline',uint8(0),'isInterrupt',uint8(0),'isChannelwise',uint8(1)),'IOBoardType',{{'DS120X','STD','ADCC1'}},'UnitType','ADC','Identifier','ADC','DialogType','ML','BlockSet','NONE','SlaveProcessor','NONE'))  RTIBlockInterface=struct('InputPortsActive',0,'InputPortsWidth',int32(1),'InputPortsDataType',{{'SS_BOOLEAN'}},'InputPortsName',{{'Continue'}},'OutputPortsActive',[1 1],'OutputPortsWidth',int32([1 1]),'OutputPortsDataType',{{'SS_DOUBLE','SS_INT16'}},'OutputPortsName',{{'ADC','Status'}},'DialogFcn','rti120xstdadcc1adcgui','SampleTime',{{-1}},'InitLevel',3,'IconTransparency','on','BlockDisplay',{{['ADC CL1\nChannel: 5'],'center'}},'BlockName',struct('Token',{{'ADC_CLASS1_BL1'}}))  RTIBlockParameters=struct('ReadMode',{{2,'OFF',[1 2]}},'ChannelNo',{{5,'OFF',[]}},'ConversionMode',{{1,'OFF',[1 2]}},'TriggerSource',{{2,'OFF',[1 2]}},'TriggerLineIn',{{1,'OFF',[1 16]}},'SampleMode',{{1,'OFF',[1 2]}},'BurstTriggerSource',{{1,'OFF',[1 2]}},'BurstTriggerLine',{{1,'OFF',[1 16]}},'ConvTriggerSource',{{3,'OFF',[1 3]}},'ConvTriggerLine',{{1,'OFF',[1 16]}},'ConvPeriod',{{'100e-6','OFF',[1e-6 1.34]}},'ConvPeriodCheck',{{0,'OFF',[]}},'BurstSize',{{'10','OFF',[]}},'BurstSizeCheck',{{0,'OFF',[]}},'DataSetOffset',{{'0','OFF',[]}},'DataSetOffsetCheck',{{0,'OFF',[]}},'DataSetLength',{{'1','OFF',[]}},'DataSetLengthCheck',{{0,'OFF',[]}},'EnableTriggerEvent',{{0,'OFF',[0 1]}},'TriggerMode',{{2,'OFF',[1 3]}},'TriggerLineOut',{{1,'OFF',[1 16]}},'ADCSWStartEnable',{{0,'OFF',[0 1]}},'SampleTime',{{'-1','OFF',[-1 inf]}},'SampleTimeCheck',{{0,'OFF',[]}},'StatusPortEnable',{{1,'OFF',[0 1]}},'TLCFileName',{{'rti120xadc_c1_adc','OFF',[]}})  RTISFcnParameters=struct('ReadMode','int16','ChannelNo','int16','ConversionMode','int16','TriggerSource','int16','TriggerLineIn','int16','SampleMode','int16','BurstTriggerSource','int16','BurstTriggerLine','int16','ConvTriggerSource','int16','ConvTriggerLine','int16','ConvPeriod','double','BurstSize','int16','DataSetOffset','int16','DataSetLength','int16','EnableTriggerEvent','int16','TriggerMode','int16','TriggerLineOut','int16','ADCSWStartEnable','int16','SampleTime','double','StatusPortEnable','int16','TLCFileName','char')  RTIBlockParaDefault=struct('ReadMode',1,'ChannelNo',1,'ConversionMode',1,'TriggerSource',1,'TriggerLineIn',1,'SampleMode',1,'BurstTriggerSource',1,'BurstTriggerLine',1,'ConvTriggerSource',3,'ConvTriggerLine',1,'ConvPeriod',0.0001,'ConvPeriodCheck',0,'BurstSize',10,'BurstSizeCheck',0,'DataSetOffset',0,'DataSetOffsetCheck',0,'DataSetLength',1,'DataSetLengthCheck',0,'EnableTriggerEvent',0,'TriggerMode',2,'TriggerLineOut',1,'ADCSWStartEnable',0,'SampleTime',-1,'SampleTimeCheck',1,'StatusPortEnable',0,'TLCFileName','rti120xadc_c1_adc')
  ADC_CLASS1_BL6 : rti1202lib_adc_class1/ADC_CLASS1_BL1  DSProperties=struct('RTI',struct('Version',uint32(1),'BlockType',struct('isSLSource',uint8(1),'isSLSink',uint8(1),'isHWSource',uint8(0),'isHWSink',uint8(1),'isSetup',uint8(0),'isInline',uint8(1),'isNonInline',uint8(0),'isInterrupt',uint8(0),'isChannelwise',uint8(1)),'IOBoardType',{{'DS120X','STD','ADCC1'}},'UnitType','ADC','Identifier','ADC','DialogType','ML','BlockSet','NONE','SlaveProcessor','NONE'))  RTIBlockInterface=struct('InputPortsActive',0,'InputPortsWidth',int32(1),'InputPortsDataType',{{'SS_BOOLEAN'}},'InputPortsName',{{'Continue'}},'OutputPortsActive',[1 1],'OutputPortsWidth',int32([1 1]),'OutputPortsDataType',{{'SS_DOUBLE','SS_INT16'}},'OutputPortsName',{{'ADC','Status'}},'DialogFcn','rti120xstdadcc1adcgui','SampleTime',{{-1}},'InitLevel',3,'IconTransparency','on','BlockDisplay',{{['ADC CL1\nChannel: 6'],'center'}},'BlockName',struct('Token',{{'ADC_CLASS1_BL1'}}))  RTIBlockParameters=struct('ReadMode',{{2,'OFF',[1 2]}},'ChannelNo',{{6,'OFF',[]}},'ConversionMode',{{1,'OFF',[1 2]}},'TriggerSource',{{2,'OFF',[1 2]}},'TriggerLineIn',{{1,'OFF',[1 16]}},'SampleMode',{{1,'OFF',[1 2]}},'BurstTriggerSource',{{1,'OFF',[1 2]}},'BurstTriggerLine',{{1,'OFF',[1 16]}},'ConvTriggerSource',{{3,'OFF',[1 3]}},'ConvTriggerLine',{{1,'OFF',[1 16]}},'ConvPeriod',{{'100e-6','OFF',[1e-6 1.34]}},'ConvPeriodCheck',{{0,'OFF',[]}},'BurstSize',{{'10','OFF',[]}},'BurstSizeCheck',{{0,'OFF',[]}},'DataSetOffset',{{'0','OFF',[]}},'DataSetOffsetCheck',{{0,'OFF',[]}},'DataSetLength',{{'1','OFF',[]}},'DataSetLengthCheck',{{0,'OFF',[]}},'EnableTriggerEvent',{{0,'OFF',[0 1]}},'TriggerMode',{{2,'OFF',[1 3]}},'TriggerLineOut',{{1,'OFF',[1 16]}},'ADCSWStartEnable',{{0,'OFF',[0 1]}},'SampleTime',{{'-1','OFF',[-1 inf]}},'SampleTimeCheck',{{0,'OFF',[]}},'StatusPortEnable',{{1,'OFF',[0 1]}},'TLCFileName',{{'rti120xadc_c1_adc','OFF',[]}})  RTISFcnParameters=struct('ReadMode','int16','ChannelNo','int16','ConversionMode','int16','TriggerSource','int16','TriggerLineIn','int16','SampleMode','int16','BurstTriggerSource','int16','BurstTriggerLine','int16','ConvTriggerSource','int16','ConvTriggerLine','int16','ConvPeriod','double','BurstSize','int16','DataSetOffset','int16','DataSetLength','int16','EnableTriggerEvent','int16','TriggerMode','int16','TriggerLineOut','int16','ADCSWStartEnable','int16','SampleTime','double','StatusPortEnable','int16','TLCFileName','char')  RTIBlockParaDefault=struct('ReadMode',1,'ChannelNo',1,'ConversionMode',1,'TriggerSource',1,'TriggerLineIn',1,'SampleMode',1,'BurstTriggerSource',1,'BurstTriggerLine',1,'ConvTriggerSource',3,'ConvTriggerLine',1,'ConvPeriod',0.0001,'ConvPeriodCheck',0,'BurstSize',10,'BurstSizeCheck',0,'DataSetOffset',0,'DataSetOffsetCheck',0,'DataSetLength',1,'DataSetLengthCheck',0,'EnableTriggerEvent',0,'TriggerMode',2,'TriggerLineOut',1,'ADCSWStartEnable',0,'SampleTime',-1,'SampleTimeCheck',1,'StatusPortEnable',0,'TLCFileName','rti120xadc_c1_adc')
  ADC_CLASS1_BL7 : rti1202lib_adc_class1/ADC_CLASS1_BL1  DSProperties=struct('RTI',struct('Version',uint32(1),'BlockType',struct('isSLSource',uint8(1),'isSLSink',uint8(1),'isHWSource',uint8(0),'isHWSink',uint8(1),'isSetup',uint8(0),'isInline',uint8(1),'isNonInline',uint8(0),'isInterrupt',uint8(0),'isChannelwise',uint8(1)),'IOBoardType',{{'DS120X','STD','ADCC1'}},'UnitType','ADC','Identifier','ADC','DialogType','ML','BlockSet','NONE','SlaveProcessor','NONE'))  RTIBlockInterface=struct('InputPortsActive',0,'InputPortsWidth',int32(1),'InputPortsDataType',{{'SS_BOOLEAN'}},'InputPortsName',{{'Continue'}},'OutputPortsActive',[1 1],'OutputPortsWidth',int32([1 1]),'OutputPortsDataType',{{'SS_DOUBLE','SS_INT16'}},'OutputPortsName',{{'ADC','Status'}},'DialogFcn','rti120xstdadcc1adcgui','SampleTime',{{-1}},'InitLevel',3,'IconTransparency','on','BlockDisplay',{{['ADC CL1\nChannel: 7'],'center'}},'BlockName',struct('Token',{{'ADC_CLASS1_BL1'}}))  RTIBlockParameters=struct('ReadMode',{{2,'OFF',[1 2]}},'ChannelNo',{{7,'OFF',[]}},'ConversionMode',{{1,'OFF',[1 2]}},'TriggerSource',{{2,'OFF',[1 2]}},'TriggerLineIn',{{1,'OFF',[1 16]}},'SampleMode',{{1,'OFF',[1 2]}},'BurstTriggerSource',{{1,'OFF',[1 2]}},'BurstTriggerLine',{{1,'OFF',[1 16]}},'ConvTriggerSource',{{3,'OFF',[1 3]}},'ConvTriggerLine',{{1,'OFF',[1 16]}},'ConvPeriod',{{'100e-6','OFF',[1e-6 1.34]}},'ConvPeriodCheck',{{0,'OFF',[]}},'BurstSize',{{'10','OFF',[]}},'BurstSizeCheck',{{0,'OFF',[]}},'DataSetOffset',{{'0','OFF',[]}},'DataSetOffsetCheck',{{0,'OFF',[]}},'DataSetLength',{{'1','OFF',[]}},'DataSetLengthCheck',{{0,'OFF',[]}},'EnableTriggerEvent',{{0,'OFF',[0 1]}},'TriggerMode',{{2,'OFF',[1 3]}},'TriggerLineOut',{{1,'OFF',[1 16]}},'ADCSWStartEnable',{{0,'OFF',[0 1]}},'SampleTime',{{'-1','OFF',[-1 inf]}},'SampleTimeCheck',{{0,'OFF',[]}},'StatusPortEnable',{{1,'OFF',[0 1]}},'TLCFileName',{{'rti120xadc_c1_adc','OFF',[]}})  RTISFcnParameters=struct('ReadMode','int16','ChannelNo','int16','ConversionMode','int16','TriggerSource','int16','TriggerLineIn','int16','SampleMode','int16','BurstTriggerSource','int16','BurstTriggerLine','int16','ConvTriggerSource','int16','ConvTriggerLine','int16','ConvPeriod','double','BurstSize','int16','DataSetOffset','int16','DataSetLength','int16','EnableTriggerEvent','int16','TriggerMode','int16','TriggerLineOut','int16','ADCSWStartEnable','int16','SampleTime','double','StatusPortEnable','int16','TLCFileName','char')  RTIBlockParaDefault=struct('ReadMode',1,'ChannelNo',1,'ConversionMode',1,'TriggerSource',1,'TriggerLineIn',1,'SampleMode',1,'BurstTriggerSource',1,'BurstTriggerLine',1,'ConvTriggerSource',3,'ConvTriggerLine',1,'ConvPeriod',0.0001,'ConvPeriodCheck',0,'BurstSize',10,'BurstSizeCheck',0,'DataSetOffset',0,'DataSetOffsetCheck',0,'DataSetLength',1,'DataSetLengthCheck',0,'EnableTriggerEvent',0,'TriggerMode',2,'TriggerLineOut',1,'ADCSWStartEnable',0,'SampleTime',-1,'SampleTimeCheck',1,'StatusPortEnable',0,'TLCFileName','rti120xadc_c1_adc')
  ADC_CLASS1_BL8 : rti1202lib_adc_class1/ADC_CLASS1_BL1  DSProperties=struct('RTI',struct('Version',uint32(1),'BlockType',struct('isSLSource',uint8(1),'isSLSink',uint8(1),'isHWSource',uint8(0),'isHWSink',uint8(1),'isSetup',uint8(0),'isInline',uint8(1),'isNonInline',uint8(0),'isInterrupt',uint8(0),'isChannelwise',uint8(1)),'IOBoardType',{{'DS120X','STD','ADCC1'}},'UnitType','ADC','Identifier','ADC','DialogType','ML','BlockSet','NONE','SlaveProcessor','NONE'))  RTIBlockInterface=struct('InputPortsActive',0,'InputPortsWidth',int32(1),'InputPortsDataType',{{'SS_BOOLEAN'}},'InputPortsName',{{'Continue'}},'OutputPortsActive',[1 1],'OutputPortsWidth',int32([1 1]),'OutputPortsDataType',{{'SS_DOUBLE','SS_INT16'}},'OutputPortsName',{{'ADC','Status'}},'DialogFcn','rti120xstdadcc1adcgui','SampleTime',{{-1}},'InitLevel',3,'IconTransparency','on','BlockDisplay',{{['ADC CL1\nChannel: 8'],'center'}},'BlockName',struct('Token',{{'ADC_CLASS1_BL1'}}))  RTIBlockParameters=struct('ReadMode',{{2,'OFF',[1 2]}},'ChannelNo',{{8,'OFF',[]}},'ConversionMode',{{1,'OFF',[1 2]}},'TriggerSource',{{2,'OFF',[1 2]}},'TriggerLineIn',{{1,'OFF',[1 16]}},'SampleMode',{{1,'OFF',[1 2]}},'BurstTriggerSource',{{1,'OFF',[1 2]}},'BurstTriggerLine',{{1,'OFF',[1 16]}},'ConvTriggerSource',{{3,'OFF',[1 3]}},'ConvTriggerLine',{{1,'OFF',[1 16]}},'ConvPeriod',{{'100e-6','OFF',[1e-6 1.34]}},'ConvPeriodCheck',{{0,'OFF',[]}},'BurstSize',{{'10','OFF',[]}},'BurstSizeCheck',{{0,'OFF',[]}},'DataSetOffset',{{'0','OFF',[]}},'DataSetOffsetCheck',{{0,'OFF',[]}},'DataSetLength',{{'1','OFF',[]}},'DataSetLengthCheck',{{0,'OFF',[]}},'EnableTriggerEvent',{{0,'OFF',[0 1]}},'TriggerMode',{{2,'OFF',[1 3]}},'TriggerLineOut',{{1,'OFF',[1 16]}},'ADCSWStartEnable',{{0,'OFF',[0 1]}},'SampleTime',{{'-1','OFF',[-1 inf]}},'SampleTimeCheck',{{0,'OFF',[]}},'StatusPortEnable',{{1,'OFF',[0 1]}},'TLCFileName',{{'rti120xadc_c1_adc','OFF',[]}})  RTISFcnParameters=struct('ReadMode','int16','ChannelNo','int16','ConversionMode','int16','TriggerSource','int16','TriggerLineIn','int16','SampleMode','int16','BurstTriggerSource','int16','BurstTriggerLine','int16','ConvTriggerSource','int16','ConvTriggerLine','int16','ConvPeriod','double','BurstSize','int16','DataSetOffset','int16','DataSetLength','int16','EnableTriggerEvent','int16','TriggerMode','int16','TriggerLineOut','int16','ADCSWStartEnable','int16','SampleTime','double','StatusPortEnable','int16','TLCFileName','char')  RTIBlockParaDefault=struct('ReadMode',1,'ChannelNo',1,'ConversionMode',1,'TriggerSource',1,'TriggerLineIn',1,'SampleMode',1,'BurstTriggerSource',1,'BurstTriggerLine',1,'ConvTriggerSource',3,'ConvTriggerLine',1,'ConvPeriod',0.0001,'ConvPeriodCheck',0,'BurstSize',10,'BurstSizeCheck',0,'DataSetOffset',0,'DataSetOffsetCheck',0,'DataSetLength',1,'DataSetLengthCheck',0,'EnableTriggerEvent',0,'TriggerMode',2,'TriggerLineOut',1,'ADCSWStartEnable',0,'SampleTime',-1,'SampleTimeCheck',1,'StatusPortEnable',0,'TLCFileName','rti120xadc_c1_adc')
  Bus Creator4 : BusCreator  Inputs=3
  Bus Creator6 : BusCreator  Inputs=12
  Gain{,1..7,12,22..29} (17 alike) : Gain
  Gain{8..11} (4 alike) : Gain  Gain=6
  Gain{13..18,20..21} (8 alike) : Gain  Gain=10
  Ground{,1..7} (8 alike) : Ground
  Sum10 : Sum  Inputs=|+-
  Sum11 : Sum  Inputs=|+-
  Sum9 : Sum  Inputs=|+-
  Terminator{,1..16} (17 alike) : Terminator
  i_c_offset : Constant  Value=-0.13
  "volt->amp_i_a           " : Gain  Gain=-12
  volt->amp_i_b : Gain  Gain=-12
  volt->amp_i_c : Gain  Gain=-12
  i(a,b,c)[A] : Outport  VectorParamsAs1DForOutWhenUnconnected=off
  AD_values[V] : Outport  Port=2  VectorParamsAs1DForOutWhenUnconnected=off
  wires:
  Gain18/1 -> Bus Creator6/10, volt->amp_i_c/1  "Voltage ADC7[V]"
  Gain17/1 -> Bus Creator6/7, volt->amp_i_b/1  "Voltage ADC5[V]"
  Gain13/1 -> Bus Creator6/1, "volt->amp_i_a           "/1  "Voltage ADC1[V]"
  "volt->amp_i_a           "/1 -> Sum9/1
  volt->amp_i_b/1 -> Sum10/1
  volt->amp_i_c/1 -> Sum11/1
  Sum11/1 -> Bus Creator4/3  "current Phase C [A]"
  Sum10/1 -> Bus Creator4/2  "current Phase B [A]"
  Sum9/1 -> Bus Creator4/1  "current Phase A [A]"
  i_c_offset/1 -> Sum11/2
  " i_a_offset"/1 -> Sum9/2
  " i_b_offset  "/1 -> Sum10/2
  Gain21/1 -> Gain11/1, Bus Creator6/11  "Voltage ADC8[V]"
  Bus Creator4/1 -> i(a,b,c)[A]/1
  Gain15/1 -> Bus Creator6/4, Gain9/1  "Voltage ADC3[V]"
  Gain14/1 -> Bus Creator6/2, Gain8/1  "Voltage ADC2[V]"
  Gain16/1 -> Gain12/1, Bus Creator6/6  "Voltage ADC4[V]"
  Gain20/1 -> Gain10/1, Bus Creator6/8  "Voltage ADC6[V]"
  Bus Creator6/1 -> AD_values[V]/1
  Gain/1 -> Terminator/1
  Ground/1 -> Gain/1  "Overflow_ADC1"
  Ground1/1 -> Gain1/1  "Overflow_ADC5"
  Gain1/1 -> Terminator1/1
  Ground2/1 -> Gain2/1  "Overflow_ADC7"
  Gain2/1 -> Terminator2/1
  Ground3/1 -> Gain3/1  "Overflow_ADC2"
  Gain3/1 -> Terminator3/1
  Ground4/1 -> Gain4/1  "Overflow_ADC3"
  Gain4/1 -> Terminator4/1
  Ground5/1 -> Gain5/1  "Overflow_ADC4"
  Gain5/1 -> Terminator5/1
  Ground6/1 -> Gain6/1  "Overflow_ADC6"
  Gain6/1 -> Terminator6/1
  Ground7/1 -> Gain7/1  "Overflow_ADC8"
  Gain7/1 -> Terminator7/1
  Gain8/1 -> Bus Creator6/3  "PhaseA_Voltage[V]"
  Gain10/1 -> Bus Creator6/9  "PhaseB_Voltage[V]"
  Gain11/1 -> Bus Creator6/12  "PhaseC_Voltage[V]"
  Gain9/1 -> Bus Creator6/5  "Battery_Voltage[V]"
  Gain12/1 -> Terminator12/1  "not_used"
  ADC_CLASS1_BL1/1 -> Gain13/1
  ADC_CLASS1_BL2/1 -> Gain14/1
  ADC_CLASS1_BL3/1 -> Gain15/1
  ADC_CLASS1_BL4/1 -> Gain16/1
  ADC_CLASS1_BL5/1 -> Gain17/1
  ADC_CLASS1_BL7/1 -> Gain18/1
  ADC_CLASS1_BL6/1 -> Gain20/1
  ADC_CLASS1_BL8/1 -> Gain21/1
  Gain22/1 -> Terminator8/1
  Gain23/1 -> Terminator9/1
  Gain24/1 -> Terminator10/1
  Gain25/1 -> Terminator11/1
  Gain26/1 -> Terminator13/1
  Gain27/1 -> Terminator14/1
  Gain28/1 -> Terminator15/1
  Gain29/1 -> Terminator16/1
  ADC_CLASS1_BL8/2 -> Gain29/1
  ADC_CLASS1_BL6/2 -> Gain28/1
  ADC_CLASS1_BL4/2 -> Gain27/1
  ADC_CLASS1_BL3/2 -> Gain26/1
  ADC_CLASS1_BL2/2 -> Gain25/1
  ADC_CLASS1_BL7/2 -> Gain24/1
  ADC_CLASS1_BL5/2 -> Gain23/1  "ADC_CL1_CH5_Status"
  ADC_CLASS1_BL1/2 -> Gain22/1  "ADC_CL1_CH1_Status"

== system PMSM_DemoBackup/Control/Input/DISCRETE_PT1 ==
  Reset[0|1] : Inport
  In : Inport  Port=2
  K : Inport  Port=3
  T[s] : Inport  Port=4
  T_Sample[s] : Inport  Port=5
  1|FilterTime : Product  Inputs=*/  InputSameDT=on  SaturateOnIntegerOverflow=on  OutDataTypeStr=Inherit: Same as first input
  Proportional : Product  Inputs=**  InputSameDT=on  SaturateOnIntegerOverflow=on  OutDataTypeStr=Inherit: Same as first input
  Sum : Sum  Inputs=-+|  InputSameDT=on  SaturateOnIntegerOverflow=on  OutDataTypeStr=Inherit: Same as first input
  Unit Delay : UnitDelay  SampleTime=-1  HasFrameUpgradeWarning=on
  discrete_Integrator_Init : Subsystem  mask(DISCRETE_INTEGRATOR){upper_limit=upper_limit_int, lower_limit=lower_limit_int, ASMProperties=struct('Name','discrete_integrator','Version','1.0','Library','ASM_ElectricComponents_lib')}
      mask prompts: upper_limit "upper limit"; lower_limit "lower limit"
      mask help: (c) Copyright 2007, dSPACE GmbH. All rights reserved.
      mask Help: eval(['asm_modelhelp(gcbh)'])
  zero : Constant  Value=0  SampleTime=-1
  Out : Outport  VectorParamsAs1DForOutWhenUnconnected=off
  wires:
  In/1 -> Proportional/1
  Sum/1 -> discrete_Integrator_Init/2(In)
  K/1 -> Proportional/2
  Proportional/1 -> Sum/2
  discrete_Integrator_Init/1(Out) -> 1|FilterTime/1
  1|FilterTime/1 -> Out/1, Unit Delay/1
  Unit Delay/1 -> Sum/1
  T[s]/1 -> 1|FilterTime/2
  Reset[0|1]/1 -> discrete_Integrator_Init/1(Reset[0|1])
  T_Sample[s]/1 -> discrete_Integrator_Init/4(T_Sample[s])
  zero/1 -> discrete_Integrator_Init/3(Initial)

== system PMSM_DemoBackup/Control/Input/SignalCollector1 ==
  BusCreator : BusCreator  Inputs=1
  tag scope: BUS_Inputs=global
  wires:
  [BUS_PMSM_IN] -> BusCreator/1
  BusCreator/1 -> [BUS_Inputs]  "Inputs"

== system PMSM_DemoBackup/Control/Input/check_apu_sensor ==
  note: As long as the encoder has
      | not detected an index signal
      | it's signals are not valid. For this
      | time the hall signals has to be used
  inc_elec_pos : Inport
  hall_pos : Inport  Port=2
  apu_sensor : Inport  Port=3
  Switch : Switch  Threshold=1.5
  pos_out : Outport  VectorParamsAs1DForOutWhenUnconnected=off
  wires:
  hall_pos/1 -> Switch/3
  Switch/1 -> pos_out/1
  apu_sensor/1 -> Switch/2
  inc_elec_pos/1 -> Switch/1
